simulink library "Dampers_Interconnected"  (R2020a)
settings: Solver=VariableStepAuto  StartTime=0.0  StopTime=10.0  RelTol=1e-3
libraries: sm_car_lib x3
Description:
  | Component of Simscape Vehicle Templates Library
  | 
  | Copyright 2018-2020 The MathWorks, Inc.
settings Model: Creator=smiller  LastModifiedBy=smiller
settings DataIOCC: ReturnWorkspaceOutputs=off
settings DebuggingCC: ArithmeticOperatorsInVariantConditions=warning
settings SFSimCC: CustomCodeUndefinedFunction=UseInterfaceOnly

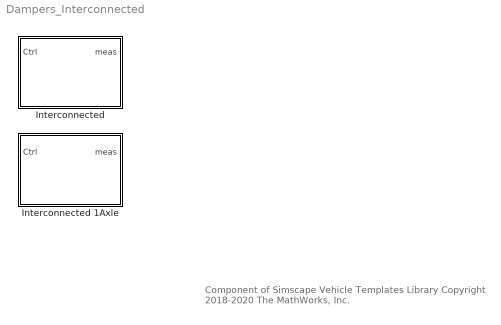
== system Dampers_Interconnected ==
  note: Component of Simscape Vehicle Templates Library
      | Copyright 2018-2020 The MathWorks, Inc.
  Interconnected : Subsystem  VariantControl=Interconnected  mask(Interconnected Dampers){InitTriggerDropdown=0}
      mask prompts: InitTriggerDropdown "Initialization Trigger Dropdown"
      mask help: Dampers connected across an axle.
      mask init:
      | curblk = gcb;
      | 
      | % Trigger Mask Initialization for 
      | % variant subsystems below this level
      | sm_car_lib_maskInitTrigger(curblk);
      mask TypeOptions InitTriggerDropdown: 0 | 1
  Interconnected 1Axle : Subsystem  VariantControl=Interconnected  mask(Interconnected Dampers){InitTriggerDropdown=0}
      mask prompts: InitTriggerDropdown "Initialization Trigger Dropdown"
      mask help: Dampers connected across an axle.
      mask init:
      | curblk = gcb;
      | 
      | % Trigger Mask Initialization for 
      | % variant subsystems below this level
      | sm_car_lib_maskInitTrigger(curblk);
      mask TypeOptions InitTriggerDropdown: 0 | 1

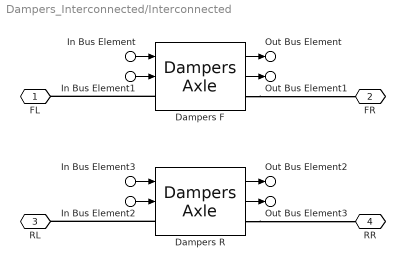
== system Dampers_Interconnected/Interconnected ==
  In Bus Element1 : Inport  PortName=Ctrl  Element=FL
  In Bus Element : Inport  PortName=Ctrl  Element=FR
  In Bus Element2 : Inport  PortName=Ctrl  Element=RL
  In Bus Element3 : Inport  PortName=Ctrl  Element=RR
  Dampers F : sm_car_lib/Springs Dampers/Dampers Axle  VariantControl=Variant1  Damper=Damper.Front  VariantLabel=Damper.Front.class.Value  InitTriggerDropdown=0
      settings: AttributesFormatString=%<ActiveVariant>
  Dampers R : sm_car_lib/Springs Dampers/Dampers Axle  VariantControl=Variant1  Damper=Damper.Rear  VariantLabel=Damper.Rear.class.Value  InitTriggerDropdown=0
      settings: AttributesFormatString=%<ActiveVariant>
  FL : PMIOPort  Side=Left
  FR : PMIOPort  Port=2  Side=Right
  RL : PMIOPort  Port=3  Side=Left
  RR : PMIOPort  Port=4  Side=Right
  Out Bus Element : Outport  VectorParamsAs1DForOutWhenUnconnected=off  PortName=meas  Element=FL
  Out Bus Element1 : Outport  VectorParamsAs1DForOutWhenUnconnected=off  PortName=meas  Element=FR
  Out Bus Element2 : Outport  VectorParamsAs1DForOutWhenUnconnected=off  PortName=meas  Element=RL
  Out Bus Element3 : Outport  VectorParamsAs1DForOutWhenUnconnected=off  PortName=meas  Element=RR
  wires:
  Dampers R/1 -> Out Bus Element2/1
  Dampers R/2 -> Out Bus Element3/1
  In Bus Element2/1 -> Dampers R/2
  In Bus Element3/1 -> Dampers R/1
  Dampers F/2 -> Out Bus Element1/1
  Dampers F/1 -> Out Bus Element/1
  In Bus Element1/1 -> Dampers F/2
  In Bus Element/1 -> Dampers F/1
  connections:
  Dampers F/RConn1 -- FR/RConn1
  Dampers F/LConn1 -- FL/RConn1
  Dampers R/RConn1 -- RR/RConn1
  Dampers R/LConn1 -- RL/RConn1

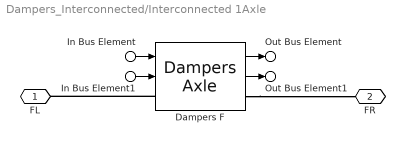
== system Dampers_Interconnected/Interconnected 1Axle ==
  In Bus Element1 : Inport  PortName=Ctrl  Element=FL
  In Bus Element : Inport  PortName=Ctrl  Element=FR
  Dampers F : sm_car_lib/Springs Dampers/Dampers Axle  VariantControl=Variant1  Damper=Damper.Front  VariantLabel=Damper.Front.class.Value  InitTriggerDropdown=0
      settings: AttributesFormatString=%<ActiveVariant>
  FL : PMIOPort  Side=Left
  FR : PMIOPort  Port=2  Side=Right
  Out Bus Element : Outport  VectorParamsAs1DForOutWhenUnconnected=off  PortName=meas  Element=FL
  Out Bus Element1 : Outport  VectorParamsAs1DForOutWhenUnconnected=off  PortName=meas  Element=FR
  wires:
  In Bus Element/1 -> Dampers F/1
  In Bus Element1/1 -> Dampers F/2
  Dampers F/1 -> Out Bus Element/1
  Dampers F/2 -> Out Bus Element1/1
  connections:
  Dampers F/LConn1 -- FL/RConn1
  Dampers F/RConn1 -- FR/RConn1
